simulink model "RTR_sim2021a_AdapSadHor"  (R2021a)
settings: Solver=ode45  StartTime=0.0  StopTime=t_stop  RelTol=1e-10
values from neighbouring files (symbols this model uses):
  Delta = 2    [RTR.m]
  g = 9.81    [RTR.m]    (also in TRT.m)
  Kd = 10    [RTR.m]
  l2 = 0.3    [RTR.m]    (also in TRT.m)
  l3 = 0.2    [RTR.m]    (also in TRT.m)
  m2 = 20    [RTR.m]    (also in TRT.m)
  m3 = 20    [RTR.m]    (also in TRT.m)
  q1_0 = 2    [RTR.m]
  q1d_0 = 0    [RTR.m]
  q1p_0 = 0    [RTR.m]
  q2_0 = 4    [RTR.m]
  q2d_0 = 1    [RTR.m]
  q2p_0 = 0    [RTR.m]
  q3_0 = 2    [RTR.m]
  q3d_0 = 0    [RTR.m]
  q3p_0 = 0    [RTR.m]
  R = 20    [RTR.m]
settings Model: Creator=kacpe  LastModifiedBy=kacpe
settings DebuggingCC: UnconnectedInputMsg=none  UnconnectedOutputMsg=none  UnconnectedLineMsg=none
settings RTWCC: DLArmComputeVersion=20.02.1

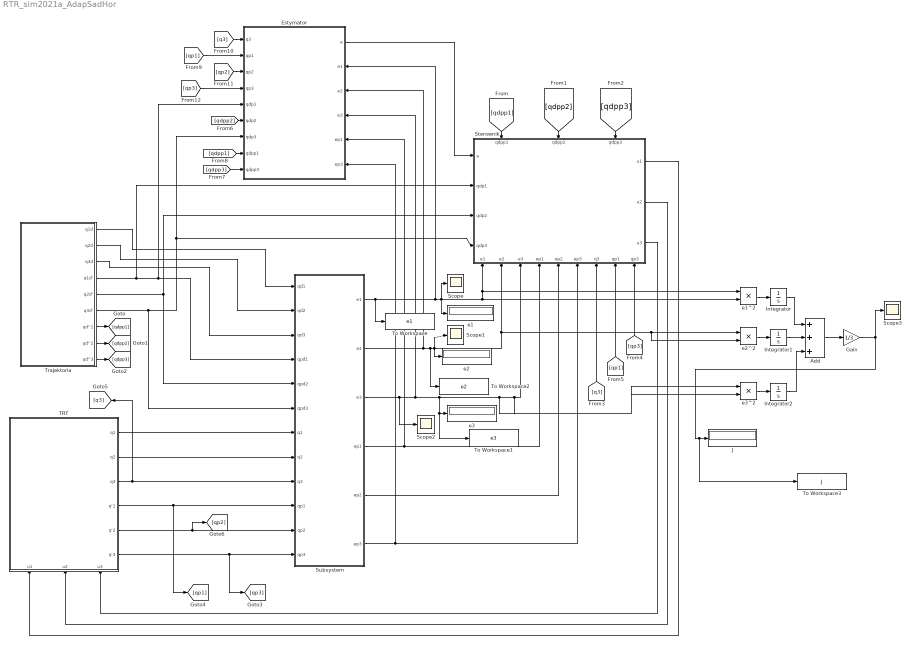
== system RTR_sim2021a_AdapSadHor ==
  Add : Sum  Inputs=+++
  Estymator : Subsystem
      settings: PortSchema="{\"entries\":[{\"content\":{\"sides\":[{\"content\":{\"connectorIds\":[\"In1\",\"In2\",\"In3\",\"In4\",\"In5\",\"In6\",\"In7\",\"In8\",\"In9\"]},\"type\":\"ConnectorPlacement.EquallySpacedRectSide\",\"uuid\":\"6cfaf714-5927-4141-bb4b-e4e1d7c7a034\"},{\"content\":{\"connectorIds\":[\"Out1\",\"In10\",\"In11\",\"In12\",\"In13\",\"In14\"],\"side\":\"RIGHT\"},\"type\":\"ConnectorPlacement.EquallySpacedRectSide\",\"uuid\":\"3cc1f1b0-216f-4715-97b4-4fb3b63e985b\"},{\"content\":{\"connectorIds\":[],\"side\":\"TOP\"},\"type\":\"ConnectorPlacement.EquallySpacedRectSide\",\"uuid\":\"9523db3e-557b-4169-8283-7761b011883a\"}]},\"type\":\"ConnectorPlacement.EquallySpacedConnector\",\"uuid\":\"a5f099c9-30c7-4e24-bbde-ab9d2a4fbad9\"}],\"packageUris\":[\"http://schema.mathworks.com/mf0/Connector/R2020b\"],\"version\":\"1.0\"}"
  Gain : Gain  Gain=1/3
  Integrator : Integrator
  Integrator1 : Integrator
  Integrator2 : Integrator
  J : Display
      settings: Format=short_e
  Scope{,1..3} (4 alike) : Scope
  Sterownik : Subsystem
      settings: PortSchema="{\"entries\":[{\"content\":{\"sides\":[{\"content\":{\"connectorIds\":[\"In1\",\"In2\",\"In3\",\"In4\"]},\"type\":\"ConnectorPlacement.EquallySpacedRectSide\",\"uuid\":\"3b6b04bd-f501-409c-86cd-e77f57a76356\"},{\"content\":{\"connectorIds\":[\"Out1\",\"Out2\",\"Out3\"],\"side\":\"RIGHT\"},\"type\":\"ConnectorPlacement.EquallySpacedRectSide\",\"uuid\":\"169b3e08-ed10-485c-953a-d5cdf046a8f4\"},{\"content\":{\"connectorIds\":[\"In5\",\"In6\",\"In7\"],\"side\":\"TOP\"},\"type\":\"ConnectorPlacement.EquallySpacedRectSide\",\"uuid\":\"f51aca33-9f1b-439e-9dc9-f4e714695a31\"},{\"content\":{\"connectorIds\":[\"In8\",\"In9\",\"In10\",\"In11\",\"In12\",\"In13\",\"In14\",\"In15\",\"In16\"],\"side\":\"BOTTOM\"},\"type\":\"ConnectorPlacement.EquallySpacedRectSide\",\"uuid\":\"22f3ba2b-e9da-4a81-be36-89fea004bef5\"}]},\"type\":\"ConnectorPlacement.EquallySpacedConnector\",\"uuid\":\"638cfe08-3a05-426d-b4bd-478b7bfa8251\"}],\"packageUris\":[\"http://schema.mathworks.com/mf0/Connector/R2020b\"],\"version\":\"1.0\"}"
  Subsystem : Subsystem
  TRT : Subsystem
      settings: PortSchema="{\"entries\":[{\"content\":{\"sides\":[{\"content\":{\"connectorIds\":[]},\"type\":\"ConnectorPlacement.EquallySpacedRectSide\",\"uuid\":\"a13a475c-743e-4b68-af9c-5e746e266b9c\"},{\"content\":{\"connectorIds\":[\"Out1\",\"Out2\",\"Out3\",\"Out4\",\"Out5\",\"Out6\"],\"side\":\"RIGHT\"},\"type\":\"ConnectorPlacement.EquallySpacedRectSide\",\"uuid\":\"c38df9ec-cc79-4f7b-9920-87d5ccf64580\"},{\"content\":{\"connectorIds\":[],\"side\":\"TOP\"},\"type\":\"ConnectorPlacement.EquallySpacedRectSide\",\"uuid\":\"3e71a422-c3ba-4d07-a3dd-6a096f4f70e7\"},{\"content\":{\"connectorIds\":[\"In1\",\"In2\",\"In3\"],\"side\":\"BOTTOM\"},\"type\":\"ConnectorPlacement.EquallySpacedRectSide\",\"uuid\":\"943e58bb-edab-4cbf-b22e-e260512a1992\"}]},\"type\":\"ConnectorPlacement.EquallySpacedConnector\",\"uuid\":\"0ec18b1f-6af6-4411-842f-55149c10a846\"}],\"packageUris\":[\"http://schema.mathworks.com/mf0/Connector/R2020b\"],\"version\":\"1.0\"}"
  To Workspace : ToWorkspace  VariableName=e1  SampleTime=-1
  To Workspace1 : ToWorkspace  VariableName=e3  SampleTime=-1
  To Workspace2 : ToWorkspace  VariableName=e2  SampleTime=-1
  To Workspace3 : ToWorkspace  VariableName=J  SampleTime=-1
  Trajektoria : Subsystem
  e1 : Display
      settings: Format=short_e
  e1^2 : Product
  e2 : Display
      settings: Format=short_e
  e2^2 : Product
  e3 : Display
      settings: Format=short_e
  e3^2 : Product
  wires:
  Trajektoria/1(q1d) -> Subsystem/1(qd1)
  Trajektoria/2(q2d) -> Subsystem/2(qd2)
  Trajektoria/3(q3d) -> Subsystem/3(qd3)
  Trajektoria/4(q1d') -> Subsystem/4(qpd1), Estymator/5(qdp1), Sterownik/2(qdp1)
  Trajektoria/5(q2d') -> Sterownik/3(qdp2), Subsystem/5(qpd2)
  Trajektoria/6(q3d') -> Sterownik/4(qdp3), Estymator/7(qdp3), Subsystem/6(qpd3)
  TRT/1(q1) -> Subsystem/7(q1)
  TRT/5(q'2) -> [qp2], Subsystem/11(qp2)
  TRT/6(q'3) -> [qp3], Subsystem/12(qp3)
  Trajektoria/7(qd''1) -> [qdpp1]
  Trajektoria/8(qd''2) -> [qdpp2]
  Trajektoria/9(qd''3) -> [qdpp3]
  [qdpp3] -> Sterownik/7(qdpp3)
  [qdpp2] -> Sterownik/6(qdpp2)
  [qdpp1] -> Sterownik/5(qdpp1)
  Subsystem/1(e1) -> To Workspace/1, Estymator/10(e1), e1/1, Scope/1, e1^2/2, e1^2/1, Sterownik/8(e1)
  Subsystem/3(e3) -> e3^2/1, e3^2/2, Sterownik/10(e3), To Workspace1/1, e3/1, Estymator/12(e3), Scope2/1
  Subsystem/4(ep1) -> Estymator/13(ep1), Sterownik/11(ep1)
  Subsystem/5(ep2) -> Sterownik/12(ep2)
  Subsystem/6(ep3) -> Estymator/14(ep3), Sterownik/13(ep3)
  TRT/4(q'1) -> [qp1], Subsystem/10(qp1)
  [q3] -> Sterownik/14(q3)
  [qp1] -> Sterownik/15(qp1)
  TRT/2(q2) -> Subsystem/8(q2)
  [qp3] -> Sterownik/16(qp3)
  Sterownik/1(u1) -> TRT/1(u1)
  Sterownik/2(u2) -> TRT/2(u2)
  Sterownik/3(u3) -> TRT/3(u3)
  [qdpp1] -> Estymator/8(qdpp1)
  [qdpp3] -> Estymator/9(qdpp3)
  [qp1] -> Estymator/2(qp1)
  [q3] -> Estymator/1(q3)
  [qp2] -> Estymator/3(qp2)
  [qp3] -> Estymator/4(qp3)
  TRT/3(q3) -> [q3], Subsystem/9(q3)
  Estymator/1(a) -> Sterownik/1(a)
  [qdpp2] -> Estymator/6(qdp2)
  e1^2/1 -> Integrator/1
  e2^2/1 -> Integrator1/1
  e3^2/1 -> Integrator2/1
  Integrator/1 -> Add/1
  Integrator1/1 -> Add/2
  Integrator2/1 -> Add/3
  Add/1 -> Gain/1
  Gain/1 -> To Workspace3/1, J/1, Scope3/1
  Subsystem/2(e2) -> Estymator/11(e2), To Workspace2/1, e2/1, Sterownik/9(e2), e2^2/2, e2^2/1, Scope1/1

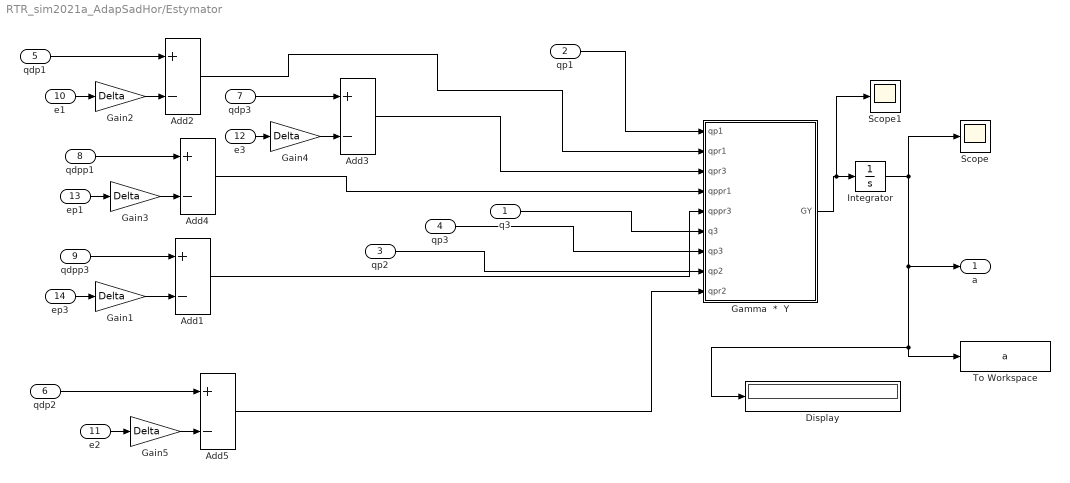
== system RTR_sim2021a_AdapSadHor/Estymator ==
  q3 : Inport
  qp1 : Inport  Port=2
  qp2 : Inport  Port=3
  qp3 : Inport  Port=4
  qdp1 : Inport  Port=5
  qdp2 : Inport  Port=6
  qdp3 : Inport  Port=7
  qdpp1 : Inport  Port=8
  qdpp3 : Inport  Port=9
  e1 : Inport  Port=10
  e2 : Inport  Port=11
  e3 : Inport  Port=12
  ep1 : Inport  Port=13
  ep3 : Inport  Port=14
  Add{1..5} (5 alike) : Sum  Inputs=+-
  Display : Display
  Gain{1..5} (5 alike) : Gain  Gain=Delta
  Gamma  *  Y : MATLAB Function  TreatAsAtomicUnit=on
  Integrator : Integrator
  Scope : Scope
  Scope1 : Scope
  To Workspace : ToWorkspace  VariableName=a  SampleTime=-1
  a : Outport
  wires:
  q3/1 -> Gamma  *  Y/6(q3)
  qdpp1/1 -> Add4/1
  ep1/1 -> Gain3/1
  Gain3/1 -> Add4/2
  Add4/1 -> Gamma  *  Y/4(qppr1)
  qdpp3/1 -> Add1/1
  Gain1/1 -> Add1/2
  ep3/1 -> Gain1/1
  Add1/1 -> Gamma  *  Y/5(qppr3)
  qdp1/1 -> Add2/1
  Gain2/1 -> Add2/2
  qdp3/1 -> Add3/1
  Gain4/1 -> Add3/2
  Add2/1 -> Gamma  *  Y/2(qpr1)
  e3/1 -> Gain4/1
  e1/1 -> Gain2/1
  Add3/1 -> Gamma  *  Y/3(qpr3)
  qp3/1 -> Gamma  *  Y/7(qp3)
  qp1/1 -> Gamma  *  Y/1(qp1)
  Gamma  *  Y/1(GY) -> Scope1/1, Integrator/1
  Integrator/1 -> To Workspace/1, Display/1, a/1, Scope/1
  qdp2/1 -> Add5/1
  Gain5/1 -> Add5/2
  e2/1 -> Gain5/1
  Add5/1 -> Gamma  *  Y/9(qpr2)
  qp2/1 -> Gamma  *  Y/8(qp2)

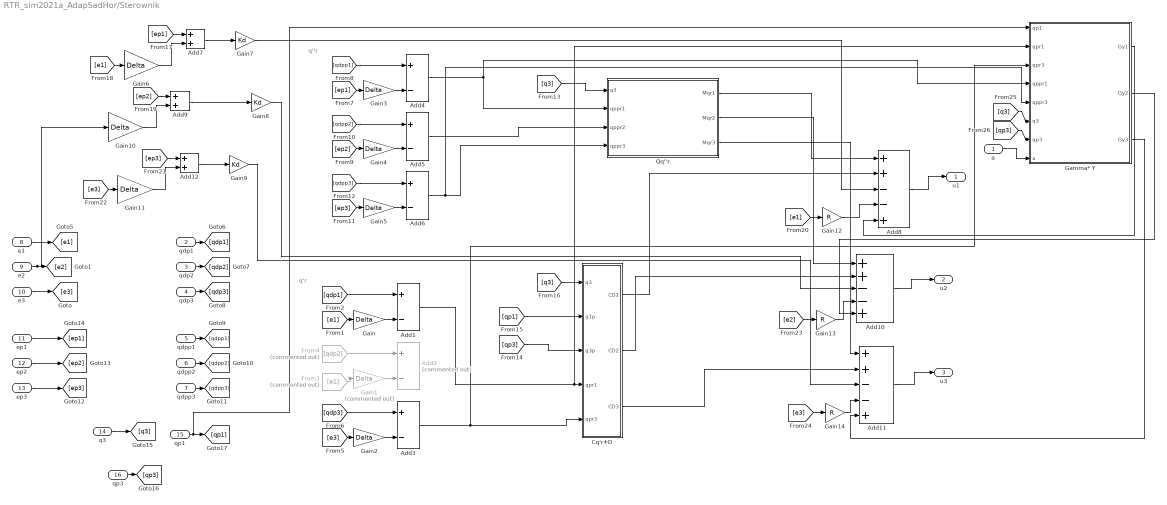
== system RTR_sim2021a_AdapSadHor/Sterownik ==
  note: q'r
  note: q''r
  a : Inport
  qdp1 : Inport  Port=2
  qdp2 : Inport  Port=3
  qdp3 : Inport  Port=4
  qdpp1 : Inport  Port=5
  qdpp2 : Inport  Port=6
  qdpp3 : Inport  Port=7
  e1 : Inport  Port=8
  e2 : Inport  Port=9
  e3 : Inport  Port=10
  ep1 : Inport  Port=11
  ep2 : Inport  Port=12
  ep3 : Inport  Port=13
  q3 : Inport  Port=14
  qp1 : Inport  Port=15
  qp3 : Inport  Port=16
  Add{1,3..6} (5 alike) : Sum  Inputs=+-
  Add10 : Sum  Inputs=++--+
  Add11 : Sum  Inputs=++--+
  Add12 : Sum
  Add2 : Sum  Commented=on  Inputs=+-
  Add7 : Sum
  Add8 : Sum  Inputs=++--+
  Add9 : Sum
  Cq'r+D : Subsystem
  From3 : From  Commented=on  GotoTag=e1
  From4 : From  Commented=on  GotoTag=qdp2
  Gain{,2..6,10..11} (8 alike) : Gain  Gain=Delta
  Gain1 : Gain  Commented=on  Gain=Delta
  Gain12 : Gain  Gain=R
  Gain13 : Gain  Gain=R
  Gain14 : Gain  Gain=R
  Gain7 : Gain  Gain=Kd
  Gain8 : Gain  Gain=Kd
  Gain9 : Gain  Gain=Kd
  Gamma* Y : MATLAB Function  TreatAsAtomicUnit=on
  Qq''r : Subsystem
  u1 : Outport
  u2 : Outport  Port=2
  u3 : Outport  Port=3
  wires:
  e3/1 -> [e3]
  e1/1 -> [e1]
  qdp1/1 -> [qdp1]
  qdp2/1 -> [qdp2]
  qdp3/1 -> [qdp3]
  qdpp1/1 -> [qdpp1]
  qdpp2/1 -> [qdpp2]
  qdpp3/1 -> [qdpp3]
  ep1/1 -> [ep1]
  ep2/1 -> [ep2]
  ep3/1 -> [ep3]
  Gain/1 -> Add1/2
  [e1] -> Gain/1
  [qdp1] -> Add1/1
  From4/1 -> Add2/1
  Gain1/1 -> Add2/2
  From3/1 -> Gain1/1
  [qdp3] -> Add3/1
  Gain2/1 -> Add3/2
  [e3] -> Gain2/1
  Add3/1 -> Gamma* Y/3(qpr3), Cq'r+D/5(qpr3)
  Add6/1 -> Gamma* Y/5(qppr3), Qq''r/4(qppr3)
  [qdpp1] -> Add4/1
  [qdpp2] -> Add5/1
  Gain3/1 -> Add4/2
  [ep1] -> Gain3/1
  Gain4/1 -> Add5/2
  Add5/1 -> Qq''r/3(qppr2)
  [ep3] -> Gain5/1
  [ep2] -> Gain4/1
  Gain5/1 -> Add6/2
  [qdpp3] -> Add6/1
  Add4/1 -> Gamma* Y/4(qppr1), Qq''r/2(qppr1)
  [q3] -> Qq''r/1(q3)
  q3/1 -> [q3]
  qp1/1 -> Gamma* Y/1(qp1), [qp1]
  qp3/1 -> [qp3]
  Add1/1 -> Gamma* Y/2(qpr1), Cq'r+D/4(qpr1)
  [qp3] -> Cq'r+D/3(q3p)
  [qp1] -> Cq'r+D/2(q1p)
  [q3] -> Cq'r+D/1(q3)
  Gain6/1 -> Add7/2
  Add7/1 -> Gain7/1
  Add9/1 -> Gain8/1
  Add12/1 -> Gain9/1
  Qq''r/1(Mqr1) -> Add8/1
  Qq''r/2(Mqr2) -> Add10/1
  Qq''r/3(Mqr3) -> Add11/1
  Cq'r+D/1(CD1) -> Add8/2
  Cq'r+D/2(CD2) -> Add10/2
  Cq'r+D/3(CD3) -> Add11/2
  Add8/1 -> u1/1
  Add10/1 -> u2/1
  Add11/1 -> u3/1
  Gain7/1 -> Add8/3
  Gain8/1 -> Add10/3
  Gain9/1 -> Add11/3
  [ep1] -> Add7/1
  [e1] -> Gain6/1
  [ep2] -> Add9/1
  e2/1 -> [e2], Gain10/1
  Gain10/1 -> Add9/2
  [ep3] -> Add12/1
  [e3] -> Gain11/1
  Gain11/1 -> Add12/2
  [e1] -> Gain12/1
  Gain12/1 -> Add8/4
  [e2] -> Gain13/1
  Gain13/1 -> Add10/4
  [e3] -> Gain14/1
  Gain14/1 -> Add11/4
  Gamma* Y/3(Gy3) -> Add11/5
  a/1 -> Gamma* Y/8(a)
  [q3] -> Gamma* Y/6(q3)
  [qp3] -> Gamma* Y/7(qp3)
  Gamma* Y/1(Gy1) -> Add8/5
  Gamma* Y/2(Gy2) -> Add10/5

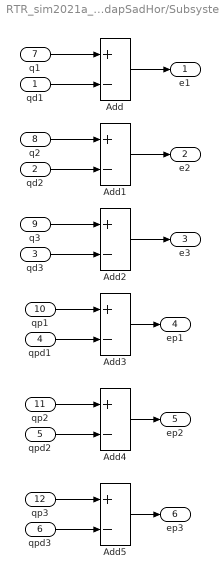
== system RTR_sim2021a_AdapSadHor/Subsystem ==
  qd1 : Inport
  qd2 : Inport  Port=2
  qd3 : Inport  Port=3
  qpd1 : Inport  Port=4
  qpd2 : Inport  Port=5
  qpd3 : Inport  Port=6
  q1 : Inport  Port=7
  q2 : Inport  Port=8
  q3 : Inport  Port=9
  qp1 : Inport  Port=10
  qp2 : Inport  Port=11
  qp3 : Inport  Port=12
  Add{,1..5} (6 alike) : Sum  Inputs=+-
  e1 : Outport
  e2 : Outport  Port=2
  e3 : Outport  Port=3
  ep1 : Outport  Port=4
  ep2 : Outport  Port=5
  ep3 : Outport  Port=6
  wires:
  qd1/1 -> Add/2
  q1/1 -> Add/1
  Add/1 -> e1/1
  q2/1 -> Add1/1
  Add1/1 -> e2/1
  qd2/1 -> Add1/2
  q3/1 -> Add2/1
  Add2/1 -> e3/1
  qd3/1 -> Add2/2
  qp1/1 -> Add3/1
  Add3/1 -> ep1/1
  qpd1/1 -> Add3/2
  qpd2/1 -> Add4/2
  qp2/1 -> Add4/1
  Add4/1 -> ep2/1
  qpd3/1 -> Add5/2
  qp3/1 -> Add5/1
  Add5/1 -> ep3/1

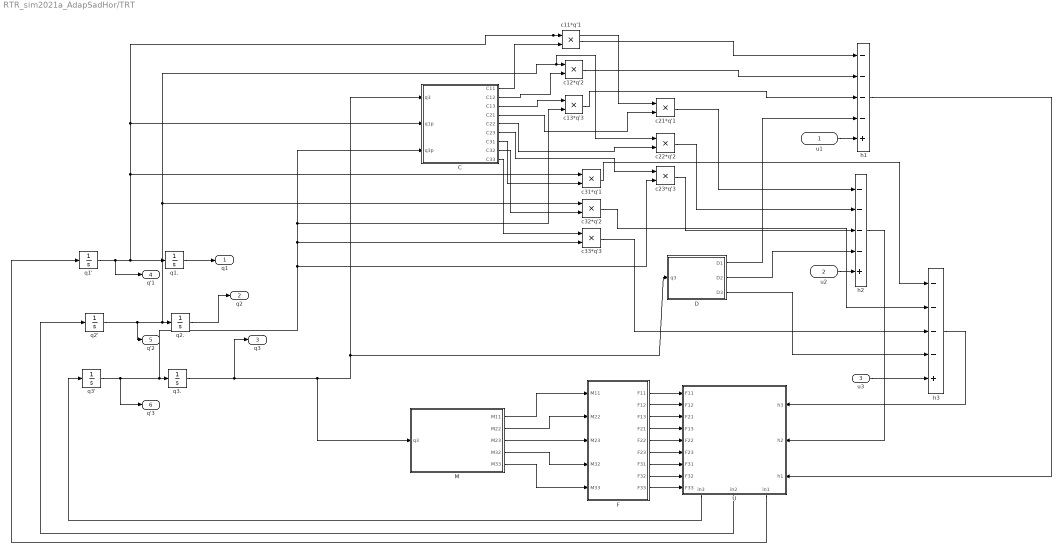
== system RTR_sim2021a_AdapSadHor/TRT ==
  u1 : Inport
  u2 : Inport  Port=2
  u3 : Inport  Port=3
  C : MATLAB Function  TreatAsAtomicUnit=on
  D : MATLAB Function  TreatAsAtomicUnit=on
  F : MATLAB Function  TreatAsAtomicUnit=on
  M : MATLAB Function  TreatAsAtomicUnit=on
  U : Subsystem
      settings: PortSchema="{\"entries\":[{\"content\":{\"sides\":[{\"content\":{\"connectorIds\":[\"In1\",\"In2\",\"In3\",\"In4\",\"In5\",\"In6\",\"In7\",\"In8\",\"In9\"]},\"type\":\"ConnectorPlacement.EquallySpacedRectSide\",\"uuid\":\"30710644-9e06-400a-91a1-da9eb46b634c\"},{\"content\":{\"connectorIds\":[\"In10\",\"In11\",\"In12\"],\"side\":\"RIGHT\"},\"type\":\"ConnectorPlacement.EquallySpacedRectSide\",\"uuid\":\"450ad47e-e867-455a-81bd-6c2cfcae7014\"},{\"content\":{\"connectorIds\":[],\"side\":\"TOP\"},\"type\":\"ConnectorPlacement.EquallySpacedRectSide\",\"uuid\":\"643bf25a-a07b-40c2-a683-349b443eb128\"},{\"content\":{\"connectorIds\":[\"Out1\",\"Out2\",\"Out3\"],\"side\":\"BOTTOM\"},\"type\":\"ConnectorPlacement.EquallySpacedRectSide\",\"uuid\":\"d7f5c48e-8c7d-4ef3-916e-98a783992e6d\"}]},\"type\":\"ConnectorPlacement.EquallySpacedConnector\",\"uuid\":\"b943515b-cd98-4c69-abf8-9cc1eb7ce306\"}],\"packageUris\":[\"http://schema.mathworks.com/mf0/Connector/R2020b\"],\"version\":\"1.0\"}"
  c11*q'1 : Product
  c12*q'2 : Product
  c13*q'3 : Product
  c21*q'1 : Product
  c22*q'2 : Product
  c23*q'3 : Product
  c31*q'1 : Product
  c32*q'2 : Product
  c33*q'3 : Product
  h1 : Sum  Inputs=----+
  h2 : Sum  Inputs=----+
  h3 : Sum  Inputs=----+
  q1' : Integrator  InitialCondition=q1p_0
  q1. : Integrator  InitialCondition=q1_0
  q2' : Integrator  InitialCondition=q2p_0
  q2. : Integrator  InitialCondition=q2_0
  q3' : Integrator  InitialCondition=q3p_0
  q3. : Integrator  InitialCondition=q3_0
  q1 : Outport
  q2 : Outport  Port=2
  q3 : Outport  Port=3
  q'1 : Outport  Port=4
  q'2 : Outport  Port=5
  q'3 : Outport  Port=6
  wires:
  M/1(M11) -> F/1(M11)
  M/2(M22) -> F/2(M22)
  M/3(M23) -> F/3(M23)
  M/4(M32) -> F/4(M32)
  M/5(M33) -> F/5(M33)
  u1/1 -> h1/5
  u3/1 -> h3/5
  u2/1 -> h2/5
  q3./1 -> C/1(q3), D/1(q3), M/1(q3), q3/1
  q3'/1 -> q'3/1, c33*q'3/2, c13*q'3/2, C/3(q3p), c23*q'3/2, q3./1
  q2'/1 -> q'2/1, c32*q'2/1, c22*q'2/1, c12*q'2/1, q2./1
  q2./1 -> q2/1
  C/1(C11) -> c11*q'1/2
  C/3(C13) -> c13*q'3/1
  C/6(C23) -> c23*q'3/1
  C/7(C31) -> c31*q'1/2
  q1./1 -> q1/1
  C/2(C12) -> c12*q'2/2
  q1'/1 -> q'1/1, c21*q'1/1, c11*q'1/1, C/2(q1p), c31*q'1/1, q1./1
  C/4(C21) -> c21*q'1/2
  C/5(C22) -> c22*q'2/2
  C/8(C32) -> c32*q'2/2
  C/9(C33) -> c33*q'3/1
  c11*q'1/1 -> h1/1
  c12*q'2/1 -> h1/2
  c13*q'3/1 -> h1/3
  D/1(D1) -> h1/4
  D/2(D2) -> h2/4
  c21*q'1/1 -> h2/1
  c22*q'2/1 -> h2/2
  D/3(D3) -> h3/4
  c31*q'1/1 -> h3/1
  c32*q'2/1 -> h3/2
  c33*q'3/1 -> h3/3
  F/1(F11) -> U/1(F11)
  F/2(F12) -> U/2(F12)
  F/3(F13) -> U/3(F21)
  F/4(F21) -> U/4(F13)
  F/5(F22) -> U/5(F22)
  F/6(F23) -> U/6(F23)
  F/7(F31) -> U/7(F31)
  F/8(F32) -> U/8(F32)
  F/9(F33) -> U/9(F33)
  h1/1 -> U/12(h1)
  h2/1 -> U/11(h2)
  h3/1 -> U/10(h3)
  U/1(in3) -> q3'/1
  U/2(in2) -> q2'/1
  U/3(in1) -> q1'/1
  c23*q'3/1 -> h2/3

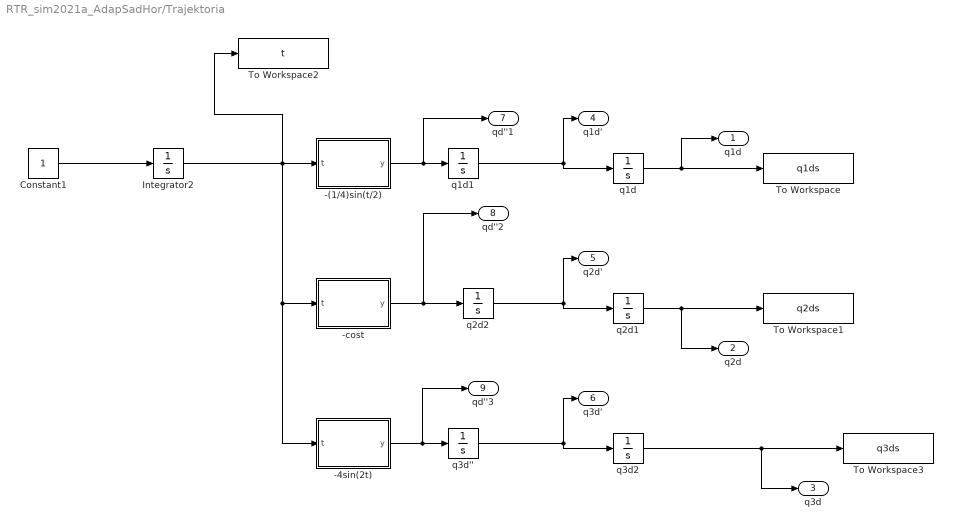
== system RTR_sim2021a_AdapSadHor/Trajektoria ==
  " q1d" : Integrator  InitialCondition=q1d_0
  " q1d1" : Integrator
  " q2d1" : Integrator  InitialCondition=q2d_0
  " q2d2" : Integrator  InitialCondition=2
  " q3d''" : Integrator
  " q3d2" : Integrator  InitialCondition=q3d_0
  -(1/4)sin(t/2) : MATLAB Function  TreatAsAtomicUnit=on
  -4sin(2t) : MATLAB Function  TreatAsAtomicUnit=on
  -cost : MATLAB Function  TreatAsAtomicUnit=on
  Constant1 : Constant
  Integrator2 : Integrator
  To Workspace : ToWorkspace  VariableName=q1ds  SampleTime=-1
  To Workspace1 : ToWorkspace  VariableName=q2ds  SampleTime=-1
  To Workspace2 : ToWorkspace  VariableName=t  SampleTime=-1
  To Workspace3 : ToWorkspace  VariableName=q3ds  SampleTime=-1
  q1d : Outport
  q2d : Outport  Port=2
  q3d : Outport  Port=3
  q1d' : Outport  Port=4
  q2d' : Outport  Port=5
  q3d' : Outport  Port=6
  qd''1 : Outport  Port=7
  qd''2 : Outport  Port=8
  qd''3 : Outport  Port=9
  wires:
  " q2d1"/1 -> To Workspace1/1, q2d/1
  -cost/1(y) -> qd''2/1, " q2d2"/1
  " q1d"/1 -> To Workspace/1, q1d/1
  -(1/4)sin(t/2)/1(y) -> qd''1/1, " q1d1"/1
  Constant1/1 -> Integrator2/1
  Integrator2/1 -> To Workspace2/1, -4sin(2t)/1(t), -cost/1(t), -(1/4)sin(t/2)/1(t)
  " q3d2"/1 -> To Workspace3/1, q3d/1
  -4sin(2t)/1(y) -> qd''3/1, " q3d''"/1
  " q3d''"/1 -> " q3d2"/1, q3d'/1
  " q2d2"/1 -> " q2d1"/1, q2d'/1
  " q1d1"/1 -> " q1d"/1, q1d'/1

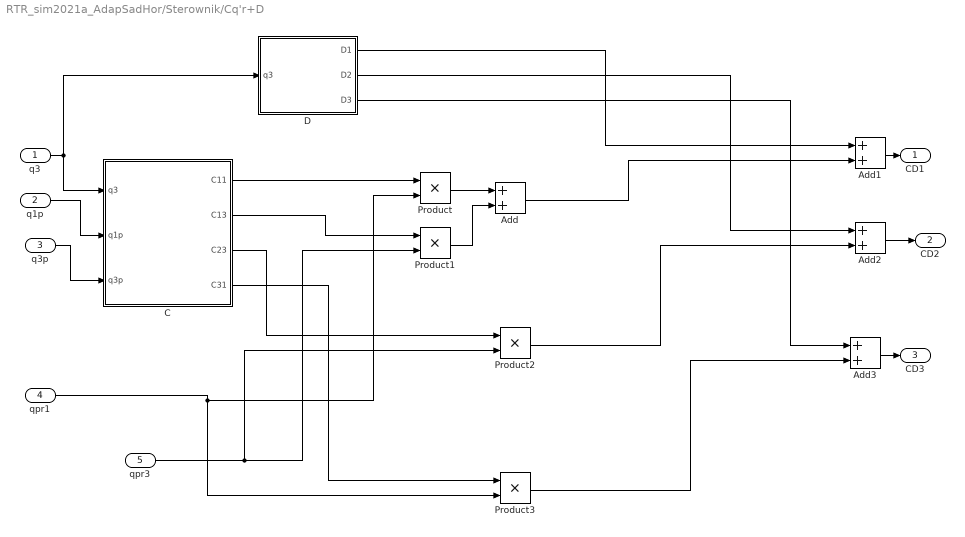
== system RTR_sim2021a_AdapSadHor/Sterownik/Cq'r+D ==
  q3 : Inport
  q1p : Inport  Port=2
  q3p : Inport  Port=3
  qpr1 : Inport  Port=4
  qpr3 : Inport  Port=5
  Add{,1..3} (4 alike) : Sum
  C : MATLAB Function  TreatAsAtomicUnit=on
  D : MATLAB Function  TreatAsAtomicUnit=on
  Product{,1..3} (4 alike) : Product
  CD1 : Outport
  CD2 : Outport  Port=2
  CD3 : Outport  Port=3
  wires:
  q3p/1 -> C/3(q3p)
  q1p/1 -> C/2(q1p)
  q3/1 -> D/1(q3), C/1(q3)
  C/1(C11) -> Product/1
  C/2(C13) -> Product1/1
  qpr1/1 -> Product3/2, Product/2
  qpr3/1 -> Product2/2, Product1/2
  C/3(C23) -> Product2/1
  C/4(C31) -> Product3/1
  Product/1 -> Add/1
  Product1/1 -> Add/2
  D/1(D1) -> Add1/1
  D/2(D2) -> Add2/1
  D/3(D3) -> Add3/1
  Add/1 -> Add1/2
  Product2/1 -> Add2/2
  Product3/1 -> Add3/2
  Add1/1 -> CD1/1
  Add2/1 -> CD2/1
  Add3/1 -> CD3/1

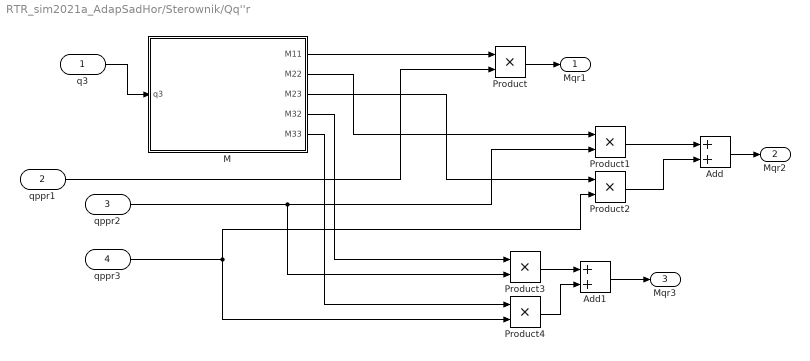
== system RTR_sim2021a_AdapSadHor/Sterownik/Qq''r ==
  q3 : Inport
  qppr1 : Inport  Port=2
  qppr2 : Inport  Port=3
  qppr3 : Inport  Port=4
  Add : Sum
  Add1 : Sum
  M : MATLAB Function  TreatAsAtomicUnit=on
  Product{,1..4} (5 alike) : Product
  Mqr1 : Outport
  Mqr2 : Outport  Port=2
  Mqr3 : Outport  Port=3
  wires:
  q3/1 -> M/1(q3)
  M/1(M11) -> Product/1
  qppr1/1 -> Product/2
  M/2(M22) -> Product1/1
  M/3(M23) -> Product2/1
  qppr2/1 -> Product3/2, Product1/2
  qppr3/1 -> Product2/2, Product4/2
  M/4(M32) -> Product3/1
  M/5(M33) -> Product4/1
  Product1/1 -> Add/1
  Product2/1 -> Add/2
  Product4/1 -> Add1/2
  Product3/1 -> Add1/1
  Product/1 -> Mqr1/1
  Add1/1 -> Mqr3/1
  Add/1 -> Mqr2/1

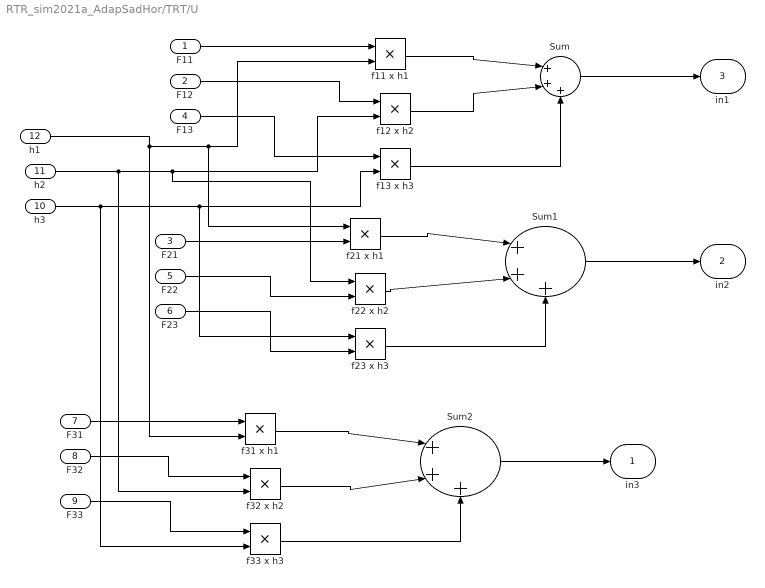
== system RTR_sim2021a_AdapSadHor/TRT/U ==
  F11 : Inport
  F12 : Inport  Port=2
  F21 : Inport  Port=3
  F13 : Inport  Port=4
  F22 : Inport  Port=5
  F23 : Inport  Port=6
  F31 : Inport  Port=7
  F32 : Inport  Port=8
  F33 : Inport  Port=9
  h3 : Inport  Port=10
  h2 : Inport  Port=11
  h1 : Inport  Port=12
  Sum : Sum  Inputs=|+++
  Sum1 : Sum  Inputs=|+++
  Sum2 : Sum  Inputs=|+++
  f11 x h1 : Product
  f12 x h2 : Product
  f13 x h3 : Product
  f21 x h1 : Product
  f22 x h2 : Product
  f23 x h3 : Product
  f31 x h1 : Product
  f32 x h2 : Product
  f33 x h3 : Product
  in3 : Outport
  in2 : Outport  Port=2
  in1 : Outport  Port=3
  wires:
  F11/1 -> f11 x h1/1
  F12/1 -> f12 x h2/1
  h2/1 -> f32 x h2/2, f22 x h2/1, f12 x h2/2
  F13/1 -> f13 x h3/1
  h3/1 -> f33 x h3/2, f23 x h3/1, f13 x h3/2
  F21/1 -> f21 x h1/2
  F22/1 -> f22 x h2/2
  F23/1 -> f23 x h3/2
  F31/1 -> f31 x h1/1
  F32/1 -> f32 x h2/1
  F33/1 -> f33 x h3/1
  h1/1 -> f31 x h1/2, f21 x h1/1, f11 x h1/2
  f11 x h1/1 -> Sum/1
  f12 x h2/1 -> Sum/2
  f13 x h3/1 -> Sum/3
  f21 x h1/1 -> Sum1/1
  f22 x h2/1 -> Sum1/2
  f23 x h3/1 -> Sum1/3
  f31 x h1/1 -> Sum2/1
  f32 x h2/1 -> Sum2/2
  f33 x h3/1 -> Sum2/3
  Sum2/1 -> in3/1
  Sum1/1 -> in2/1
  Sum/1 -> in1/1

== matlab function RTR_sim2021a_AdapSadHor/Trajektoria/-cost ==
  data: t input; y output
function y = fcn(t)

y = -cos(t);

== matlab function RTR_sim2021a_AdapSadHor/TRT/F ==
  data: M11 input; M22 input; M23 input; F11 output; M32 input; M33 input; F12 output; F13 output; F21 output; F22 output; F23 output; F31 output; F32 output; F33 output
function [F11,F12,F13,F21,F22,F23,F31,F32,F33] =fcn(M11, M22, M23, M32, M33)
%(wiersz, kolumna)
%M11, M22,  M33, M23, M32
%% output
%M=[0,0,0;0,0,0;0,0,0];
M = [M11, 0, 0;
     0, M22, M23;
     0,M32, M33];

F1 = inv(M);
F11 = F1(1,1);
F12 = F1(1,2);
F13 = F1(1,3);
F21 = F1(2,1);
F22 = F1(2,2);
F23 = F1(2,3);
F31 = F1(3,1);
F32 = F1(3,2);
F33 = F1(3,3);

== matlab function RTR_sim2021a_AdapSadHor/Sterownik/Qq''r/M ==
  data: l2 parameter; l3 parameter; m2 parameter; m3 parameter; q3 input; M11 output; M22 output; M23 output; M32 output; M33 output
function [M11, M22, M23, M32, M33] =fcn(l2,l3, m2, m3, q3)
%(wiersz, kolumna)
%M11, M22,  M33, M23, M32
%% output
%M=[0,0,0;0,0,0;0,0,0];
M11 = (1/3)*m2*(l2^2)+(m3*(l2^2)+(cos(q3)^2) + m3*l2*l3*cos(3));
M22 = m2+m3;
M23 = (1/2)*m3*l2*l3*cos(q3);
M32 = (1/2)*m3*l2*l3*cos(q3);
M33 = 0;
%M0=0;

== matlab function RTR_sim2021a_AdapSadHor/Sterownik/Cq'r+D/C ==
  data: q3 input; q1p input; q3p input; m3 parameter; l2 parameter; l3 parameter; C11 output; C13 output; C23 output; C31 output
function [C11, C13,C23, C31] =fcn( q3, q1p, q3p, m3, l2, l3)
%(wiersz, kolumna)
%M11, M22,  M33, M23, M32
%% output
%M=[0,0,0;0,0,0;0,0,0];
C11 = -q3p*((1/2)*m3*l2*l3*sin(q3) + sin(q3)*cos(q3));
C13 = -q1p*((1/2)*m3*l2*l3*sin(q3) + sin(q3)*cos(q3));
C23 = -q3p*(1/2)*m3*(l3*l2)*sin(q3)*cos(q3);
C31 = q1p*((1/2)*m3*l2*l3*sin(q3) + sin(q3)*cos(q3));
%C0 = 0;
% C12 = 0;
% C21 = 0;
% C22 = 0; 
% C32 = 0;
% C33 = 0;

== matlab function RTR_sim2021a_AdapSadHor/Sterownik/Cq'r+D/D ==
  data: q3 input; m2 parameter; m3 parameter; l3 parameter; g parameter; D1 output; D2 output; D3 output
function [D1, D2, D3] =fcn(q3,m2,m3, l3, g)
%(wiersz, kolumna)
%M11, M22,  M33, M23, M32
%% output
%M=[0,0,0;0,0,0;0,0,0];
D1 = 0;
D2 = (m2+m3)*g;
D3 = (1/2)*g*m3*l3*cos(q3);

== matlab function RTR_sim2021a_AdapSadHor/Estymator/Gamma  *  Y ==
  data: qp1 input; qpr1 input; GY output; qpr3 input; qppr1 input; qppr3 input; q3 input; qp3 input; Gamma parameter; qp2 input; qpr2 input
function GY  = fcn(qp1,qpr1,qpr3,qppr1,qppr3,q3,qp3,Gamma,qp2,qpr2)

Y11 = (cos(q3)^2)*qppr1 - sin(q3)*cos(q3)*qp3*qpr1;
Y13 = -qp1*sin(q3)*cos(q3)*qpr3;
Y31 = qp1*sin(q3)*cos(q3)*qpr1;
Y33 = qppr3;
s1 = qp1 - qpr1;
s2 = qp2 - qpr2;
s3 = qp3 - qpr3;
G = Gamma;
GY = -G *[(Y11+ Y31), 0, (Y13+ Y33)]*[s1,s2,s3]';

% GY = -G *[(Y11+ Y13), 0, (Y31+ Y33)]*[s1,s2,s3]';

== matlab function RTR_sim2021a_AdapSadHor/Sterownik/Gamma* Y ==
  data: qp1 input; qpr1 input; Gy1 output; qpr3 input; qppr1 input; qppr3 input; q3 input; qp3 input; a input; Gy2 output; Gy3 output
function [Gy1, Gy2, Gy3] = fcn(qp1,qpr1,qpr3,qppr1,qppr3,q3,qp3,a)

Y11 = (cos(q3)^2)*qppr1 - sin(q3)*cos(q3)*qp3*qpr1;
Y13 = -qp1*sin(q3)*cos(q3)*qpr3;
Y31 = qp1*sin(q3)*cos(q3)*qpr1;
Y33 = qppr3;

GY = [(Y11+ Y31), 0, (Y13+ Y33)]*a;
Gy1 = GY(1);
Gy2 = GY(2);
Gy3=GY(3);

== matlab function RTR_sim2021a_AdapSadHor/Trajektoria/-4sin(2t) ==
  data: t input; y output
function y = fcn(t)

y = -4*sin(2*t);

== matlab function RTR_sim2021a_AdapSadHor/TRT/M ==
  data: l2 parameter; l3 parameter; m2 parameter; m3 parameter; q3 input; M11 output; M22 output; M23 output; M32 output; M33 output
function [M11, M22, M23, M32, M33] =fcn(l2,l3, m2, m3, q3)
%(wiersz, kolumna)
%M11, M22,  M33, M23, M32
%% output
%M=[0,0,0;0,0,0;0,0,0];
M11 = (1/3)*m2*(l2^2)+m3*((l2^2)+(1/3)*(l3^2)*(cos(q3)^2) + l2*l3*cos(3));
M22 = m2+m3;
M23 = (1/2)*m3*l2*l3*cos(q3);
M32 = (1/2)*m3*l2*l3*cos(q3);
M33 = (1/3)*m3*(l3^2);
%M0=0;

== matlab function RTR_sim2021a_AdapSadHor/TRT/C ==
  data: q3 input; q1p input; q3p input; m3 parameter; l2 parameter; l3 parameter; C11 output; C12 output; C13 output; C21 output; C22 output; C23 output; C31 output; C32 output; C33 output
function [C11,C12, C13,C21,C22,C23, C31,C32,C33] =fcn( q3, q1p, q3p, m3, l2, l3)
%(wiersz, kolumna)
%M11, M22,  M33, M23, M32
%% output
%M=[0,0,0;0,0,0;0,0,0];
C11 = -q3p*((1/2)*m3*l2*l3*sin(q3) + (1/3)*m3*(l3^2)*sin(q3)*cos(q3));
C13 = -q1p*((1/2)*m3*l2*l3*sin(q3) + (1/3)*m3*(l3^2)*sin(q3)*cos(q3));
C23 = -q3p*(1/2)*m3*(l3*l2)*sin(q3)*cos(q3);
C31 = q1p*((1/2)*m3*l2*l3*sin(q3) + (1/3)*m3*(l3^2)*sin(q3)*cos(q3));
%C0 = 0;
C12 = 0;
C21 = 0;
C22 = 0; 
C32 = 0;
C33 = 0;

== matlab function RTR_sim2021a_AdapSadHor/TRT/D ==
  data: q3 input; m2 parameter; m3 parameter; l3 parameter; g parameter; D1 output; D2 output; D3 output
function [D1, D2, D3] =fcn(q3,m2,m3, l3, g)
%(wiersz, kolumna)
%M11, M22,  M33, M23, M32
%% output
%M=[0,0,0;0,0,0;0,0,0];
D1 = 0;
D2 = (m2+m3)*g;
D3 = (1/2)*g*m3*l3*cos(q3);

== matlab function RTR_sim2021a_AdapSadHor/Trajektoria/-(1//4)sin(t//2) ==
  data: t input; y output
function y = fcn(t)

y = -(1/4)*sin(t/2);
